simulink model "system_1"  (R2022b)
settings: Solver=VariableStepAuto  StartTime=0.0  StopTime=1  RelTol=1e-4
settings Model: Creator=Dongr  LastModifiedBy=Dongr

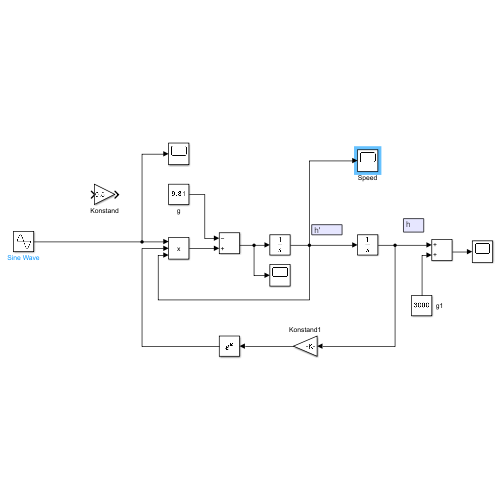
[thumbnail: Simulink's stored preview of the top-level diagram]
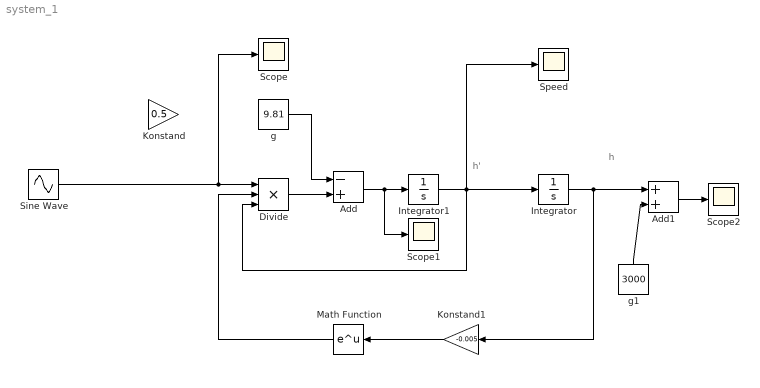
== system system_1 ==
  note: h'
  note: h
  Add : Sum  Inputs=-+
  Add1 : Sum
  Divide : Product  Inputs=***
  Integrator : Integrator
  Integrator1 : Integrator
  Konstand : Gain  Gain=0.5
  Konstand1 : Gain  Gain=-0.005
  Math Function : Math
  Scope : Scope
  Scope1 : Scope
  Scope2 : Scope
  Sine Wave : Sin  Amplitude=2  Frequency=50  Phase=30  SampleTime=0
  Speed : Scope
  g : Constant  Value=9.81
  g1 : Constant  Value=3000
  wires:
  Integrator/1 -> Konstand1/1, Add1/1
  Integrator1/1 -> Divide/3, Integrator/1, Speed/1
  Math Function/1 -> Divide/2
  Add/1 -> Scope1/1, Integrator1/1
  Divide/1 -> Add/2
  g/1 -> Add/1
  Add1/1 -> Scope2/1
  g1/1 -> Add1/2
  Sine Wave/1 -> Scope/1, Divide/1
  Konstand1/1 -> Math Function/1
